simulink model "rendezvous_model"  (R2020b)
settings: Solver=VariableStepAuto  StartTime=0.0  StopTime=10.0  RelTol=1e-3
settings Model: Creator=dipietrant  LastModifiedBy=dipietrant

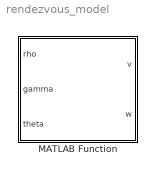
== system rendezvous_model ==
  MATLAB Function : MATLAB Function  TreatAsAtomicUnit=on

== matlab function rendezvous_model/MATLAB Function ==
  data: rho input; v output; gamma input; theta input; w output
function [v, w]= fcn(rho, gamma, theta)

v = k1 * rho*cos(gamma);
w = k2 * gamma + k1*sin(gamma)*cos(gamma)/gamma*(gamma + k3*(gamma+theta));
